simulink model "SWC_VES_type"  (R2021b)
settings: Solver=FixedStepDiscrete  StartTime=0.0  StopTime=10.0  FixedStep=0.001  RelTol=1e-3
undefined symbols (not defined in the file or in its folder): boolean_OTAMode, R_HALINCDD_CSOP_IPCF_Handler, R_VESCDD_CSOP_OTA_Mode
settings Model: DataDictionary=APPTypes.sldd  Creator=FVT23010  LastModifiedBy=FVT23010
settings DataIOCC: SaveFormat=StructureWithTime
settings OptimizationCC: DefaultParameterBehavior=Inlined  EnhancedBackFolding=on  PassReuseOutputArgsAs=Individual arguments  ZeroExternalMemoryAtStartup=off  ZeroInternalMemoryAtStartup=off  OptimizeBlockOrder=speed  DifferentSizesBufferReuse=on  OptimizationCustomize=off  EfficientTunableParamExpr=on
settings DebuggingCC: ParameterTunabilityLossMsg=error
settings ModelReferenceCC: ModelReferenceNumInstancesAllowed=Single
settings SFSimCC: MATLABDynamicMemAlloc=off
settings RTWCC: Description=AUTOSAR  SystemTargetFile=autosar.tlc  GenCodeOnly=on  TemplateMakefile=ert_default_tmf
settings CodeAppCC: ForceParamTrailComments=on  IgnoreCustomStorageClasses=off  OperatorAnnotations=on  SimulinkDataObjDesc=on  SFDataObjDesc=on  InsertBlockDesc=on
settings STFCustomTargetCC: TargetLangStandard=C99 (ISO)  MultiwordLength=256  ParMdlRefBuildCompliant=on  CompOptLevelCompliant=on  IncludeMdlTerminateFcn=off  CombineOutputUpdateFcns=on  SuppressErrorStatus=on  ERTCustomFileBanners=on  SupportNonFinite=off  SupportComplex=off  SupportContinuousTime=off  SupportNonInlinedSFcns=off  RemoveResetFunc=on  MATLABClassNameForMDSCustomization=Simulink.SoftwareTarget.ERTCustomization  AutosarCompliant=on  GRTInterface=off  UseToolchainInfoCompliant=on  LookupTableObjectStructAxisOrder=2,1,3,4,...  LUTObjectStructOrderEvenSpacing=Size,Table,Breakpoints  SystemTargetFile=autosar.tlc
settings ERTTargetCC: TargetLangStandard=C99 (ISO)  ConcurrentExecutionCompliant=off  IncludeMdlTerminateFcn=off  SuppressErrorStatus=on  SupportNonFinite=off  SupportComplex=off  ModelStepFunctionPrototypeControlCompliant=off  CPPClassGenCompliant=off  AutosarCompliant=on  LookupTableObjectStructAxisOrder=2,1,3,4,...  LUTObjectStructOrderEvenSpacing=Size,Table,Breakpoints  InlinedParameterPlacement=NonHierarchical  ERTCustomFileTemplate=example_file_process.tlc

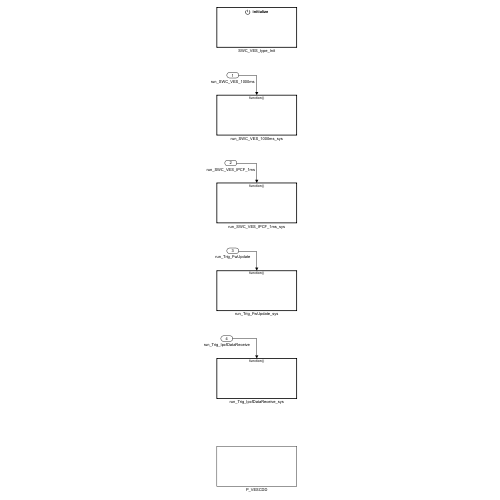
[thumbnail: Simulink's stored preview of the top-level diagram]
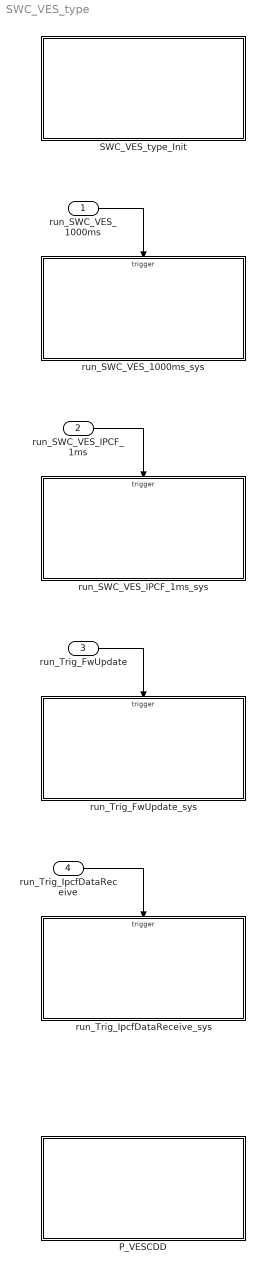
== system SWC_VES_type ==
  run_SWC_VES_1000ms : Inport  SampleTime=1  OutputFunctionCall=on
  run_SWC_VES_IPCF_1ms : Inport  Port=2  SampleTime=0.001  OutputFunctionCall=on
  run_Trig_FwUpdate : Inport  Port=3  OutputFunctionCall=on
  run_Trig_IpcfDataReceive : Inport  Port=4  OutputFunctionCall=on
  P_VESCDD : Subsystem
  SWC_VES_type_Init : Subsystem
  run_SWC_VES_1000ms_sys : Subsystem
  run_SWC_VES_IPCF_1ms_sys : Subsystem
  run_Trig_FwUpdate_sys : Subsystem
  run_Trig_IpcfDataReceive_sys : Subsystem
  wires:
  run_SWC_VES_1000ms/1 -> run_SWC_VES_1000ms_sys/Trigger
  run_SWC_VES_IPCF_1ms/1 -> run_SWC_VES_IPCF_1ms_sys/Trigger
  run_Trig_FwUpdate/1 -> run_Trig_FwUpdate_sys/Trigger
  run_Trig_IpcfDataReceive/1 -> run_Trig_IpcfDataReceive_sys/Trigger

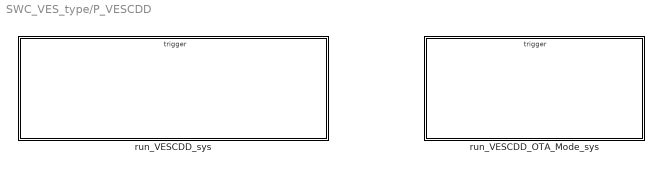
== system SWC_VES_type/P_VESCDD ==
  run_VESCDD_OTA_Mode_sys : Subsystem
  run_VESCDD_sys : Subsystem

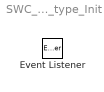
== system SWC_VES_type/SWC_VES_type_Init ==
  Event Listener : EventListener  EventName=reset

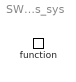
== system SWC_VES_type/run_SWC_VES_1000ms_sys ==
  function : TriggerPort  TriggerType=function-call  VariantControl=(inherit)  SampleTimeType=periodic  SampleTime=-1

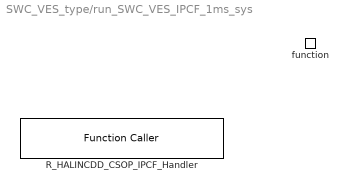
== system SWC_VES_type/run_SWC_VES_IPCF_1ms_sys ==
  function : TriggerPort  TriggerType=function-call  VariantControl=(inherit)  SampleTimeType=periodic  SampleTime=-1
  R_HALINCDD_CSOP_IPCF_Handler : FunctionCaller  FunctionPrototype=R_HALINCDD_CSOP_IPCF_Handler()

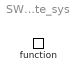
== system SWC_VES_type/run_Trig_FwUpdate_sys ==
  function : TriggerPort  TriggerType=function-call  VariantControl=(inherit)

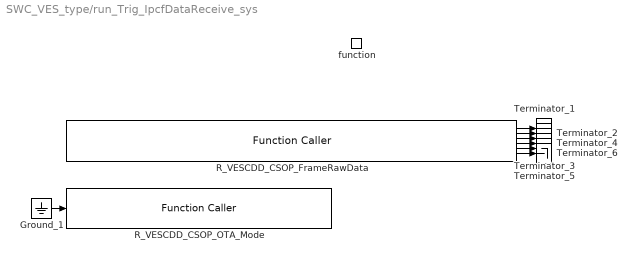
== system SWC_VES_type/run_Trig_IpcfDataReceive_sys ==
  function : TriggerPort  TriggerType=function-call  VariantControl=(inherit)
  Ground_1 : Ground
  R_VESCDD_CSOP_FrameRawData : FunctionCaller  FunctionPrototype=[channel,fd,ext,id,dlc,FrameRawData] = R_VESCDD_CSOP_FrameRawData()  OutputArgumentSpecifications=uint8(1), uint8(1), uint8(1), uint32(1), uint8(1), uint8([1;1;1;1;1;1;1;1;1;1;1;1;1;1;1;1;1;1;1;1;1;1;1;1;1;1;1;1;1;1;1;1;1;1;1;1;1;1;1;1;1;1;1;1;1;1;1;1;1;1;1;1;1;1;1;1;1;1;1;1;1;1;1;1])
  R_VESCDD_CSOP_OTA_Mode : FunctionCaller  FunctionPrototype=R_VESCDD_CSOP_OTA_Mode(boolean_OTAMode)  InputArgumentSpecifications=boolean(true)
  Terminator_{1..6} (6 alike) : Terminator
  wires:
  R_VESCDD_CSOP_FrameRawData/1 -> Terminator_1/1
  R_VESCDD_CSOP_FrameRawData/2 -> Terminator_2/1
  R_VESCDD_CSOP_FrameRawData/3 -> Terminator_3/1
  R_VESCDD_CSOP_FrameRawData/4 -> Terminator_4/1
  R_VESCDD_CSOP_FrameRawData/5 -> Terminator_5/1
  R_VESCDD_CSOP_FrameRawData/6 -> Terminator_6/1
  Ground_1/1 -> R_VESCDD_CSOP_OTA_Mode/1

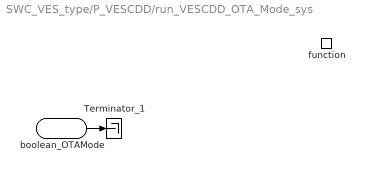
== system SWC_VES_type/P_VESCDD/run_VESCDD_OTA_Mode_sys ==
  function : TriggerPort  TriggerType=function-call  IsSimulinkFunction=on  FunctionName=run_VESCDD_OTA_Mode  VariantControl=(inherit)
  Terminator_1 : Terminator
  boolean_OTAMode : ArgIn  OutDataTypeStr=boolean  ArgumentName=boolean_OTAMode
  wires:
  boolean_OTAMode/1 -> Terminator_1/1

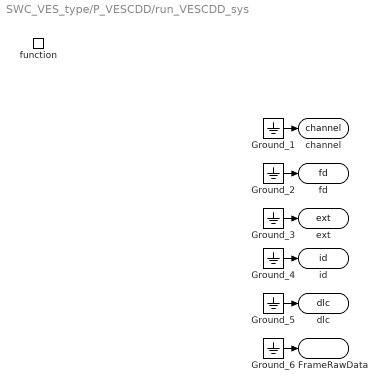
== system SWC_VES_type/P_VESCDD/run_VESCDD_sys ==
  function : TriggerPort  TriggerType=function-call  IsSimulinkFunction=on  FunctionName=run_VESCDD  VariantControl=(inherit)
  Ground_{1..6} (6 alike) : Ground
  channel : ArgOut  OutDataTypeStr=uint8  ArgumentName=channel
  fd : ArgOut  Port=2  OutDataTypeStr=uint8  ArgumentName=fd
  ext : ArgOut  Port=3  OutDataTypeStr=uint8  ArgumentName=ext
  id : ArgOut  Port=4  OutDataTypeStr=uint32  ArgumentName=id
  dlc : ArgOut  Port=5  OutDataTypeStr=uint8  ArgumentName=dlc
  FrameRawData : ArgOut  Port=6  OutDataTypeStr=uint8  PortDimensions=[64 64]  ArgumentName=FrameRawData
  wires:
  Ground_1/1 -> channel/1
  Ground_2/1 -> fd/1
  Ground_3/1 -> ext/1
  Ground_4/1 -> id/1
  Ground_5/1 -> dlc/1
  Ground_6/1 -> FrameRawData/1
